simulink model "Exercitiul3"  (R2016a)
settings: Solver=VariableStepAuto  StartTime=0.0  StopTime=28800  RelTol=1e-3
undefined symbols (not defined in the file): m, n
settings Model: Creator=Cristina  LastModifiedBy=Cristina

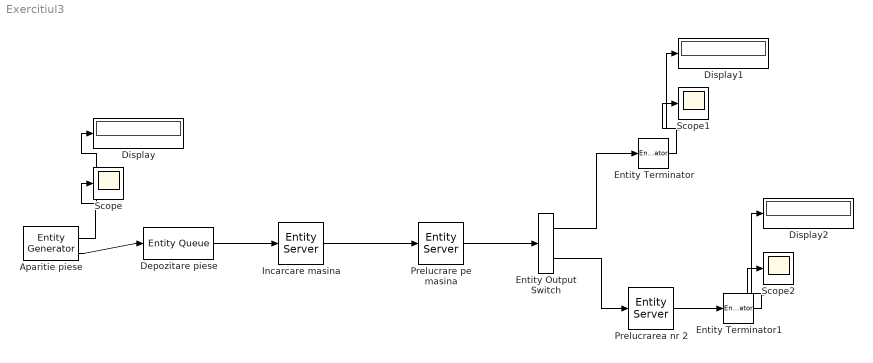
== system Exercitiul3 ==
  Aparitie piese : EntityGenerator  OutputPortMessageModes=n,m  TimeSource=MATLAB action  IntergenerationTimeAction=|  AttributeName=prt  NumberEntitiesDeparted=on  EntityType=Structured  EntityTypeName=Entity
      | persistent init
      | if (isempty(init))
      |     rng(123);
      |     init = true;
      | end
      | dt = 60 + 120 * rand;
      settings: OutputPortMap=o0,o3
  Depozitare piese : EntityQueue  InputPortMessageModes=m  OutputPortMessageModes=m
      settings: OutputPortMap=o5
  Display : Display
  Display1 : Display
  Display2 : Display
  Entity Output Switch : EntityOutputSwitch  InputPortMessageModes=m  OutputPortMessageModes=m,m  SwitchingCriterion=From attribute  SwitchAttributeName=prt
  Entity Terminator : EntityTerminator  InputPortMessageModes=m  NumberEntitiesArrived=on
      settings: OutputPortMap=o0
  Entity Terminator1 : EntityTerminator  InputPortMessageModes=m  NumberEntitiesArrived=on
      settings: OutputPortMap=o0
  Incarcare masina : EntityServer  InputPortMessageModes=m  OutputPortMessageModes=m  Capacity=1  ServiceTimeSource=MATLAB action  ServiceTimeAction=|
      | persistent init
      | if (isempty(init))
      |     rng(124);
      |     init = true;
      | end
      | dt = 40 + 40 * rand;
  "Prelucrare pe masina " : EntityServer  InputPortMessageModes=m  OutputPortMessageModes=m  Capacity=1  ServiceTimeSource=MATLAB action  ServiceTimeAction=|  EntryAction=|
      ServiceTimeAction=|
      | persistent init
      | if (isempty(init))
      |     rng(123);
      |     init = true;
      | end
      | dt = 120 + 120 * rand;
      EntryAction=|
      | if rand < 0.3
      |     entity.prt = 2;
      | else
      |     entity.prt = 1;
      | end
  Prelucrarea nr 2 : EntityServer  InputPortMessageModes=m  OutputPortMessageModes=m  Capacity=1  ServiceTimeSource=MATLAB action  ServiceTimeAction=|
      | persistent init
      | if (isempty(init))
      |     rng(125);
      |     init = true;
      | end
      | dt = 70 + 100 * rand;
  Scope : Scope
  Scope1 : Scope
  Scope2 : Scope
  wires:
  Aparitie piese/2 -> Depozitare piese/1
  Incarcare masina/1 -> "Prelucrare pe masina "/1
  "Prelucrare pe masina "/1 -> Entity Output Switch/1
  Entity Output Switch/2 -> Prelucrarea nr 2/1
  Entity Output Switch/1 -> Entity Terminator/1
  Prelucrarea nr 2/1 -> Entity Terminator1/1
  Depozitare piese/1 -> Incarcare masina/1
  Aparitie piese/1 -> Display/1, Scope/1
  Entity Terminator/1 -> Display1/1, Scope1/1
  Entity Terminator1/1 -> Display2/1, Scope2/1
